simulink model "EV_Model"  (R2020b)
settings: Solver=VariableStepAuto  StartTime=0.0  StopTime=inf  RelTol=1e-3
undefined symbols (not defined in the file): battery, DCDC, DCU, DCU1, DiscIntNeverNeededParam, ECP, HVH, magnitude, PAR, PTC, road, SampleTime, VCU, veh, wheel
libraries: simulink x10
(part 2 of 2)

== system EV_Model/Driver/DriverModel/WhlTrqCal/Fitted Drag Force  ==
  VehVelTrgt_kph : Inport
  Add : Sum  Inputs=+++
  Constant : Constant  Value=veh.RoadResistance.F0
  Constant1 : Constant  Value=veh.RoadResistance.F1
  Constant2 : Constant  Value=veh.RoadResistance.F2
  Math Function : Math  Operator=magnitude^2  SaturateOnIntegerOverflow=on
  Product : Product
  Product1 : Product
  WhlForceReq_N : Outport
  wires:
  Constant1/1 -> Product1/2
  Constant2/1 -> Product/2
  VehVelTrgt_kph/1 -> Product1/1, Math Function/1
  Math Function/1 -> Product/1
  Product/1 -> Add/1
  Product1/1 -> Add/2
  Constant/1 -> Add/3
  Add/1 -> WhlForceReq_N/1

== system EV_Model/Driver/DriverModel/WhlTrqCal/Grade Resisitance ==
  Sum2 : Sum
  g : Constant  Value=veh.Gravity
  grade resistance : Product  Inputs=***
  mass : Constant  Value=veh.Mass.Empty
  mass_refer : Constant  Value=veh.Mass.Refer
  road grade : Constant  Value=road.Grade/sqrt(road.Grade^2+1)
  GradeForce_N : Outport  VectorParamsAs1DForOutWhenUnconnected=off
  wires:
  road grade/1 -> grade resistance/3
  grade resistance/1 -> GradeForce_N/1
  g/1 -> grade resistance/2
  mass_refer/1 -> Sum2/1
  mass/1 -> Sum2/2
  Sum2/1 -> grade resistance/1

== system EV_Model/Driver/DriverModel/WhlTrqCal/PreCycle ==
  clock : Inport
  cycle_length : Inport  Port=2
  time_offset : Inport  Port=3
  Product : Product  Inputs=*/  SaturateOnIntegerOverflow=on  OutDataTypeStr=Inherit: Same as first input
  Product1 : Product  SaturateOnIntegerOverflow=on  OutDataTypeStr=Inherit: Same as first input
  Rounding Function : Rounding
  Sum1 : Sum  InputSameDT=on  SaturateOnIntegerOverflow=on  OutDataTypeStr=Inherit: Same as first input
  Sum4 : Sum  Inputs=+-  InputSameDT=on  SaturateOnIntegerOverflow=on  OutDataTypeStr=Inherit: Same as first input
  clock1 : InportShadow
  cycle_length1 : InportShadow  Port=2
  time : Outport  VectorParamsAs1DForOutWhenUnconnected=off
  wires:
  Sum1/1 -> time/1
  time_offset/1 -> Sum1/2
  Sum4/1 -> Sum1/1
  Product1/1 -> Sum4/2
  Rounding Function/1 -> Product1/1
  Product/1 -> Rounding Function/1
  cycle_length/1 -> Product/2
  clock/1 -> Product/1
  cycle_length1/1 -> Product1/2
  clock1/1 -> Sum4/1

== system EV_Model/Driver/DriverModel/WhlTrqCal/Vehicle Equivalent Mass ==
  Product1 : Product
  Sum2 : Sum
  inertia coefficient : Constant  Value=veh.InerCoeff
  mass_refer : Constant  Value=veh.Mass.Refer
  vehicle mass : Constant  Value=veh.Mass.Empty
  EquivMass_kg : Outport
  wires:
  Product1/1 -> EquivMass_kg/1
  inertia coefficient/1 -> Product1/2
  Sum2/1 -> Product1/1
  vehicle mass/1 -> Sum2/1
  mass_refer/1 -> Sum2/2

== system EV_Model/Drivetrain/Subsystem/MOTOR/Efficiency ==
  BattVolt_V : Inport
  MotTrqCmd_Nm : Inport  Port=2
  MotSpdAct_rpm : Inport  Port=3
  "Crossfade " : Subsystem  AncestorBlock=GAC_library/Crossfade  mask(Crossfade){}
      mask help: Gradual changing of output in accordance with input siganl F. When the input signal F equals MX, Out equals max. When the input signal F equals NRM, Out equals norm. When the input signal F equals MN, Out equals min. When signal F is between the nominated values of MX/NRM or MN/NRM, then output executes liner interpolation.
      mask Display:
      | color('black')
      | port_label('input', 1, 'F');
      | port_label('input', 2, 'max');
      | port_label('input', 3, 'norm');
      | port_label('input', 4, 'min');
      | port_label('input', 5, 'MX');
      | port_label('input', 6, 'NRM');
      | port_label('input', 7, 'MN');
      | port_label('output',1, 'out');
      | plot(100,100);
      | plot(0,0);
      | color('blue');
      | plot([40 70],[20 20]);
      | plot([40 70],[50 50]);
      | plot([40 70],[80 80]);
      | plot([55 55],[20 80]);
      | text(30,20,'-1');
      | text(30,50,'0');
      | text(30,80,'1');
  DCU1.EffMap(highVolt) : Lookup_n-D  BreakpointsForDimension1=DCU1.EffMap.map1.TrqTab  BreakpointsForDimension2=DCU1.EffMap.map1.SpdTab  Table=DCU1.EffMap.map1.EffTab  InternalRulePriority=Speed  RndMeth=Simplest  InputSameDT=on
      settings: InputPortMap=u0,u1
  DCU1.EffMap(lowVolt) : Lookup_n-D  BreakpointsForDimension1=DCU1.EffMap.map3.TrqTab  BreakpointsForDimension2=DCU1.EffMap.map3.SpdTab  Table=DCU1.EffMap.map3.EffTab  InternalRulePriority=Speed  RndMeth=Simplest  InputSameDT=on
      settings: InputPortMap=u0,u1
  DCU1.EffMap(mediumVolt) : Lookup_n-D  BreakpointsForDimension1=DCU1.EffMap.map2.TrqTab  BreakpointsForDimension2=DCU1.EffMap.map2.SpdTab  Table=DCU1.EffMap.map2.EffTab  InternalRulePriority=Speed  RndMeth=Simplest  InputSameDT=on
      settings: InputPortMap=u0,u1
  MATLAB Function : MATLAB Function  TreatAsAtomicUnit=on
  Saturation : Saturate  UpperLimit=1  LowerLimit=0.2
  Unit Delay : UnitDelay  SampleTime=-1  HasFrameUpgradeWarning=on
  constant1 : Constant  Value=DCU1.EffMap.map1.Volt
  constant2 : Constant  Value=DCU1.EffMap.map2.Volt
  constant3 : Constant  Value=DCU1.EffMap.map3.Volt
  MotEffi_1 : Outport  VectorParamsAs1DForOutWhenUnconnected=off
  wires:
  constant3/1 -> "Crossfade "/7(min_in)
  constant2/1 -> "Crossfade "/6("norm_in ")
  constant1/1 -> "Crossfade "/5(max_in)
  DCU1.EffMap(lowVolt)/1 -> "Crossfade "/4(min_out)
  DCU1.EffMap(mediumVolt)/1 -> "Crossfade "/3("norm_out ")
  DCU1.EffMap(highVolt)/1 -> "Crossfade "/2(max_out)
  "Crossfade "/1(Output) -> Saturation/1
  BattVolt_V/1 -> "Crossfade "/1(F_in)
  Saturation/1 -> MATLAB Function/1(u1)
  Unit Delay/1 -> MATLAB Function/2(u2)
  MATLAB Function/1(y) -> MotEffi_1/1, Unit Delay/1
  MotTrqCmd_Nm/1 -> DCU1.EffMap(highVolt)/1, DCU1.EffMap(mediumVolt)/1, DCU1.EffMap(lowVolt)/1
  MotSpdAct_rpm/1 -> DCU1.EffMap(highVolt)/2, DCU1.EffMap(mediumVolt)/2, DCU1.EffMap(lowVolt)/2

== system EV_Model/Drivetrain/Subsystem/MOTOR/MotTrqFilter ==
  MotTrqCmd_Nm : Inport
  Add1 : Sum
  Add3 : Sum
  Constant1 : Constant  Value=0.1
  Constant2 : Constant  Value=veh.MotTrqFilter
  Constant3 : Constant  Value=VCU.sampleTime
  Divide : Product  Inputs=*/
  Divide1 : Product  Inputs=/*
  Product1 : Product  RndMeth=Zero
  Product2 : Product  RndMeth=Zero
  Switch : Switch  Criteria=u2 > Threshold
  Unit Delay1 : UnitDelay  SampleTime=-1  HasFrameUpgradeWarning=on
  MotTrqCmdFilter_Nm : Outport  VectorParamsAs1DForOutWhenUnconnected=off
  wires:
  Constant1/1 -> Divide/1, Add1/1  "Tc"
  Add1/1 -> Divide/2, Divide1/1
  Constant3/1 -> Add1/2, Divide1/2  "Ts"
  Divide1/1 -> Product2/1
  MotTrqCmd_Nm/1 -> Switch/3, Product2/2
  Add3/1 -> Switch/1, Unit Delay1/1  "out"
  Divide/1 -> Product1/2
  Product1/1 -> Add3/1
  Product2/1 -> Add3/2
  Unit Delay1/1 -> Product1/1
  Switch/1 -> MotTrqCmdFilter_Nm/1
  Constant2/1 -> Switch/2

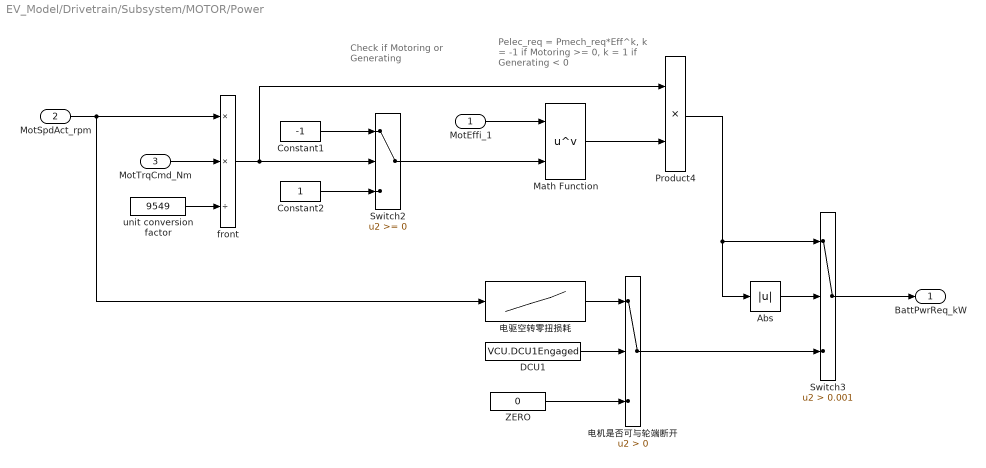
== system EV_Model/Drivetrain/Subsystem/MOTOR/Power ==
  note: Pelec_req = Pmech_req*Eff^k,
      | k = -1 if Motoring >= 0,
      | k = 1 if Generating < 0
  note: Check if Motoring
      | or Generating
  MotEffi_1 : Inport
  MotSpdAct_rpm : Inport  Port=2
  MotTrqCmd_Nm : Inport  Port=3
  Abs : Abs
  Constant1 : Constant  Value=-1  SampleTime=-1
  Constant2 : Constant  SampleTime=-1
  DCU1 : Constant  Value=VCU.DCU1Engaged
  Math Function : Math  Operator=pow  SignedPower=on  OutputSignalType=real  SaturateOnIntegerOverflow=on
  Product4 : Product
  Switch2 : Switch
  Switch3 : Switch  Criteria=u2 > Threshold  Threshold=0.001  ZeroCross=off
  "ZERO " : Constant  Value=0
  "front " : Product  Inputs=**/
  unit conversion factor : Constant  Value=9549
  电机是否可与轮端断开 : Switch  Criteria=u2 > Threshold  ZeroCross=off
  电驱空转零扭损耗 : Lookup_n-D  NumberOfTableDimensions=1  BreakpointsForDimension1=DCU1.ZeroTrqLoss.SpdTab  Table=DCU1.ZeroTrqLoss.PwrTab  InternalRulePriority=Speed  RndMeth=Simplest  InputSameDT=on
  BattPwrReq_kW : Outport  VectorParamsAs1DForOutWhenUnconnected=off
  wires:
  "ZERO "/1 -> 电机是否可与轮端断开/3
  电驱空转零扭损耗/1 -> 电机是否可与轮端断开/1
  DCU1/1 -> 电机是否可与轮端断开/2
  Switch3/1 -> BattPwrReq_kW/1
  MotSpdAct_rpm/1 -> 电驱空转零扭损耗/1, "front "/1
  Abs/1 -> Switch3/2
  unit conversion factor/1 -> "front "/3
  MotTrqCmd_Nm/1 -> "front "/2
  Constant2/1 -> Switch2/3
  Constant1/1 -> Switch2/1
  电机是否可与轮端断开/1 -> Switch3/3
  "front "/1 -> Product4/1, Switch2/2
  Switch2/1 -> Math Function/2
  MotEffi_1/1 -> Math Function/1
  Math Function/1 -> Product4/2
  Product4/1 -> Switch3/1, Abs/1

== system EV_Model/VCU/Subsystem/Batt Pwr Limit/Check Within Limits ==
  up : Inport
  u : Inport  Port=2
  lo : Inport  Port=3
  Compare To Zero : simulink/Logic and Bit Operations/Compare To Zero  relop=>=  OutDataTypeStr=boolean
  Compare To Zero1 : simulink/Logic and Bit Operations/Compare To Zero  relop=<=  OutDataTypeStr=boolean
  Logical Operator : Logic  AllPortsSameDT=off  OutDataTypeStr=boolean
  Saturation Dynamic1 : simulink/Discontinuities/Saturation Dynamic  OutMin=[]  OutMax=[]  OutDataTypeStr=Inherit: Same as second input  OutDataType=fixdt(1, 16)  OutScaling=2^-10  DoSatur=off
  Subtract : Sum  Inputs=+-
  Subtract1 : Sum  Inputs=-+
  InLimit : Outport  VectorParamsAs1DForOutWhenUnconnected=off
  y : Outport  Port=2  VectorParamsAs1DForOutWhenUnconnected=off
  wires:
  Saturation Dynamic1/1 -> y/1
  lo/1 -> Subtract1/2, Saturation Dynamic1/3
  up/1 -> Subtract/1, Saturation Dynamic1/1
  u/1 -> Subtract1/1, Subtract/2, Saturation Dynamic1/2
  Subtract/1 -> Compare To Zero/1
  Subtract1/1 -> Compare To Zero1/1
  Compare To Zero/1 -> Logical Operator/1
  Compare To Zero1/1 -> Logical Operator/2
  Logical Operator/1 -> InLimit/1

== system EV_Model/VCU/Subsystem/Mot Torque Request Cal/Series Regen Braking ==
  TrqReq_Nm : Inport
  DCUTrqLimit_Nm : Inport  Port=2
  VehSpd : Inport  Port=3
  BattSoc : Inport  Port=4
  Abs : Abs
  ChrgLmt : Lookup_n-D  NumberOfTableDimensions=1  BreakpointsForDimension1=[0 10 20 30 40 50 60 70 80 90 100]  Table=[1 1 1 1 1 1 1 1 0.7 0.35 0]  ExtrapMethod=Clip  UseLastTableValue=on  InternalRulePriority=Speed  RndMeth=Simplest  InputSameDT=on
  Gain : Gain  Gain=-1
  MinMax : MinMax  Inputs=2
  Product1 : Product
  Product3 : Product
  RegenBrakingCutoff : Lookup_n-D  NumberOfTableDimensions=1  BreakpointsForDimension1=[0 5 12 200]  Table=[0 0 1 1]  ExtrapMethod=Clip  UseLastTableValue=on  InternalRulePriority=Speed  RndMeth=Simplest  InputSameDT=on
  Saturation : Saturate  UpperLimit=0  LowerLimit=-inf
  " MotTrqRegenReq_Nm" : Outport  VectorParamsAs1DForOutWhenUnconnected=off
  wires:
  MinMax/1 -> Product3/1
  ChrgLmt/1 -> Product1/2
  VehSpd/1 -> RegenBrakingCutoff/1
  RegenBrakingCutoff/1 -> Product1/1
  Product1/1 -> Product3/2  "RegenFactor"
  BattSoc/1 -> ChrgLmt/1
  DCUTrqLimit_Nm/1 -> MinMax/2
  Product3/1 -> Gain/1
  TrqReq_Nm/1 -> Saturation/1
  Saturation/1 -> Abs/1  "DCUBrkTrqReq_Nm"
  Abs/1 -> MinMax/1
  Gain/1 -> " MotTrqRegenReq_Nm"/1

== system EV_Model/Vehicle/Dynamic/Road Ressistance/Fitted Drag Force  ==
  VehVelAct_kph : Inport
  Add : Sum  Inputs=+++
  Constant : Constant  Value=veh.RoadResistance.F0
  Constant1 : Constant  Value=veh.RoadResistance.F1
  Constant2 : Constant  Value=veh.RoadResistance.F2
  Math Function : Math  Operator=magnitude^2  SaturateOnIntegerOverflow=on
  Product : Product
  Product1 : Product
  WhlForceReq_N : Outport
  wires:
  Constant1/1 -> Product1/2
  Constant2/1 -> Product/2
  VehVelAct_kph/1 -> Product1/1, Math Function/1
  Math Function/1 -> Product/1
  Product/1 -> Add/1
  Product1/1 -> Add/2
  Constant/1 -> Add/3
  Add/1 -> WhlForceReq_N/1

== system EV_Model/Vehicle/Dynamic/Road Ressistance/Grade Resisitance ==
  Sum2 : Sum
  g : Constant  Value=veh.Gravity
  grade resistance : Product  Inputs=***
  mass : Constant  Value=veh.Mass.Empty
  mass_refer : Constant  Value=veh.Mass.Refer
  road grade : Constant  Value=road.Grade/sqrt(road.Grade^2+1)
  GradeForce_N : Outport  VectorParamsAs1DForOutWhenUnconnected=off
  wires:
  road grade/1 -> grade resistance/3
  grade resistance/1 -> GradeForce_N/1
  g/1 -> grade resistance/2
  mass_refer/1 -> Sum2/1
  mass/1 -> Sum2/2
  Sum2/1 -> grade resistance/1

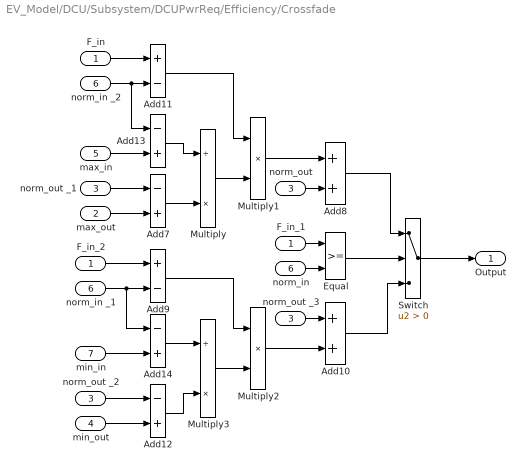
== system EV_Model/DCU/Subsystem/DCUPwrReq/Efficiency/Crossfade  ==
  F_in : Inport
  max_out : Inport  Port=2
  "norm_out " : Inport  Port=3
  min_out : Inport  Port=4
  max_in : Inport  Port=5
  "norm_in " : Inport  Port=6
  min_in : Inport  Port=7
  Add10 : Sum
  Add11 : Sum  Inputs=+-
  Add{7,12..14} (4 alike) : Sum  Inputs=-+
  Add8 : Sum
  Add9 : Sum  Inputs=+-
  Equal : RelationalOperator  OutDataTypeStr=boolean  RndMeth=Simplest
  F_in_1 : InportShadow
  F_in_2 : InportShadow
  Multiply : Product  Inputs=/*
  Multiply1 : Product  Inputs=**
  Multiply2 : Product  Inputs=**
  Multiply3 : Product  Inputs=/*
  Switch : Switch  Criteria=u2 > Threshold
  norm_in _1 : InportShadow  Port=6
  norm_in _2 : InportShadow  Port=6
  norm_out _1 : InportShadow  Port=3
  norm_out _2 : InportShadow  Port=3
  norm_out _3 : InportShadow  Port=3
  Output : Outport  VectorParamsAs1DForOutWhenUnconnected=off
  wires:
  Add11/1 -> Multiply1/1
  Add8/1 -> Switch/1
  norm_out _3/1 -> Add10/1
  Add12/1 -> Multiply3/2
  "norm_out "/1 -> Add8/2
  F_in/1 -> Add11/1
  Switch/1 -> Output/1
  Add13/1 -> Multiply/1
  norm_in _1/1 -> Add14/1, Add9/2
  Add9/1 -> Multiply2/1
  max_out/1 -> Add7/2
  norm_in _2/1 -> Add13/1, Add11/2
  max_in/1 -> Add13/2
  norm_out _1/1 -> Add7/1
  Multiply1/1 -> Add8/1
  Add7/1 -> Multiply/2
  Add10/1 -> Switch/3
  norm_out _2/1 -> Add12/1
  Multiply/1 -> Multiply1/2
  min_in/1 -> Add14/2
  Multiply3/1 -> Multiply2/2
  Multiply2/1 -> Add10/2
  "norm_in "/1 -> Equal/2
  F_in_1/1 -> Equal/1
  Equal/1 -> Switch/2
  F_in_2/1 -> Add9/1
  Add14/1 -> Multiply3/1
  min_out/1 -> Add12/2

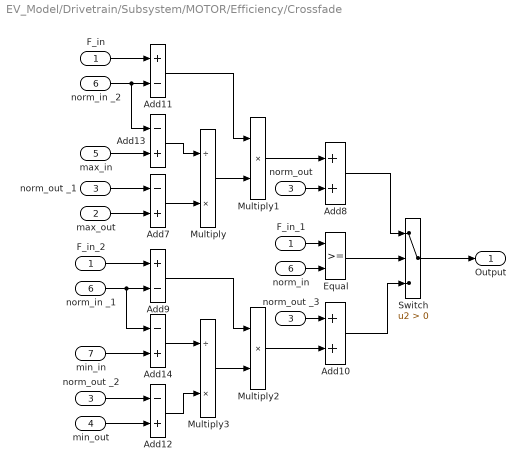
== system EV_Model/Drivetrain/Subsystem/MOTOR/Efficiency/Crossfade  ==
  F_in : Inport
  max_out : Inport  Port=2
  "norm_out " : Inport  Port=3
  min_out : Inport  Port=4
  max_in : Inport  Port=5
  "norm_in " : Inport  Port=6
  min_in : Inport  Port=7
  Add10 : Sum
  Add11 : Sum  Inputs=+-
  Add{7,12..14} (4 alike) : Sum  Inputs=-+
  Add8 : Sum
  Add9 : Sum  Inputs=+-
  Equal : RelationalOperator  OutDataTypeStr=boolean  RndMeth=Simplest
  F_in_1 : InportShadow
  F_in_2 : InportShadow
  Multiply : Product  Inputs=/*
  Multiply1 : Product  Inputs=**
  Multiply2 : Product  Inputs=**
  Multiply3 : Product  Inputs=/*
  Switch : Switch  Criteria=u2 > Threshold
  norm_in _1 : InportShadow  Port=6
  norm_in _2 : InportShadow  Port=6
  norm_out _1 : InportShadow  Port=3
  norm_out _2 : InportShadow  Port=3
  norm_out _3 : InportShadow  Port=3
  Output : Outport  VectorParamsAs1DForOutWhenUnconnected=off
  wires:
  Add11/1 -> Multiply1/1
  Add8/1 -> Switch/1
  norm_out _3/1 -> Add10/1
  Add12/1 -> Multiply3/2
  "norm_out "/1 -> Add8/2
  F_in/1 -> Add11/1
  Switch/1 -> Output/1
  Add13/1 -> Multiply/1
  norm_in _1/1 -> Add14/1, Add9/2
  Add9/1 -> Multiply2/1
  max_out/1 -> Add7/2
  norm_in _2/1 -> Add13/1, Add11/2
  max_in/1 -> Add13/2
  norm_out _1/1 -> Add7/1
  Multiply1/1 -> Add8/1
  Add7/1 -> Multiply/2
  Add10/1 -> Switch/3
  norm_out _2/1 -> Add12/1
  Multiply/1 -> Multiply1/2
  min_in/1 -> Add14/2
  Multiply3/1 -> Multiply2/2
  Multiply2/1 -> Add10/2
  "norm_in "/1 -> Equal/2
  F_in_1/1 -> Equal/1
  Equal/1 -> Switch/2
  F_in_2/1 -> Add9/1
  Add14/1 -> Multiply3/1
  min_out/1 -> Add12/2

== matlab function EV_Model/Drivetrain/Subsystem/MOTOR/Efficiency/MATLAB Function ==
  data: u1 input; y output; u2 input
function y = fcn(u1,u2)
if isnan(u1)
    y = u2;
else
    y = u1;
end

== matlab function EV_Model/DCU/Subsystem/DCUPwrReq/Efficiency/MATLAB Function ==
  data: u1 input; y output; u2 input
function y = fcn(u1,u2)
if isnan(u1)
    y = u2;
else
    y = u1;
end
